simulink model "STEP3"  (R2020b)
settings: Solver=FixedStepDiscrete  StartTime=0.0  StopTime=inf  FixedStep=1  RelTol=1e-3  EnableMultiTasking=on
PreLoadFcn:
  | defaultRadioRequestMode = RadioRequestMode.OFF;
  | defaultCdRequestMode = CdRequestMode.EMPTY;
StartFcn:
  | clear sfcdplayerhelper;
  | sfcdplayergui;
StopFcn:
  | delete(sfcdplayergui);
model workspace (MATLAB code in the model file):
  | Ts = 0.01;  % setup system sample rate
settings Model: Creator=The MathWorks, Inc.  LastModifiedBy=Fong
settings DataIOCC: LimitDataPoints=on  SaveFormat=Array  SaveOutput=off  SaveTime=off  ReturnWorkspaceOutputs=off
settings OptimizationCC: DefaultParameterBehavior=Inlined  ExpressionDepthLimit=2147483647  StateBitsets=on  DataBitsets=on  ZeroExternalMemoryAtStartup=off  ZeroInternalMemoryAtStartup=off  InitFltsAndDblsToZero=on  EfficientFloat2IntCast=on  EfficientMapNaN2IntZero=off  LifeSpan=1  EfficientTunableParamExpr=on
settings DebuggingCC: UnderspecifiedInitializationDetection=Classic  MergeDetectMultiDrivingBlocksExec=none  FcnCallInpInsideContextMsg=warning  AllowSymbolicDim=off  StateNameClashWarn=warning  SFUnexpectedBacktrackingDiag=warning  SFNoUnconditionalDefaultTransitionDiag=warning  SFExecutionAtInitializationDiag=none  ArithmeticOperatorsInVariantConditions=warning
settings HardwareCC: ProdBitPerPointer=32  ProdBitPerSizeT=32  ProdBitPerPtrDiffT=32  ProdLargestAtomicFloat=None  ProdWordSize=32  ProdHWDeviceType=NEC->V850
settings ModelReferenceCC: ModelReferenceNumInstancesAllowed=Single  PropagateSignalLabelsOutOfModel=off
settings SFSimCC: SimUseLocalCustomCode=off  SimParseCustomCode=off  CustomCodeUndefinedFunction=UseInterfaceOnly
settings RTWCC: Description=Real-Time Workshop Embedded Coder (no auto configuration)  SystemTargetFile=ert.tlc  GenCodeOnly=on  TemplateMakefile=ert_default_tmf  GenerateReport=on  RTWUseLocalCustomCode=off  IncludeHyperlinkInReport=on  LaunchReport=on  GenerateTraceInfo=on  GenerateTraceReport=on  GenerateTraceReportSl=on  GenerateTraceReportSf=on  GenerateTraceReportEml=on
settings CodeAppCC: IgnoreCustomStorageClasses=off  CustomSymbolStrType=$N$R$M  CustomSymbolStrModelFcn=$N  StateflowObjectComments=on  InternalIdentifier=Classic
settings ERTTargetCC: MultiwordLength=2048  GenerateSampleERTMain=on  IncludeMdlTerminateFcn=off  SupportAbsoluteTime=off  PurelyIntegerCode=on  SupportNonFinite=off  SupportComplex=off  ERTCustomFileTemplate=example_file_process.tlc  ConvertIfToSwitch=off  SuppressUnreachableDefaultCases=off  EnableUserReplacementTypes=on
settings ConfigComp: CovMetricSettings=dw  CovSaveCumulativeToWorkspaceVar=on  CovSaveSingleToWorkspaceVar=on  CovExternalEMLEnable=off  CovSFcnEnable=off  DVMaxProcessTime=600  DVParameters=on  DVModelCoverageObjectives=MCDC  DVMaxTestCaseSteps=500  DVTestSuiteOptimization=CombinedObjectives  DVDetectActiveLogic=on  DVSaveHarnessModel=on  DVModelReferenceHarness=on  DVSaveReport=on  DVRebuildModelRepresentation=Always

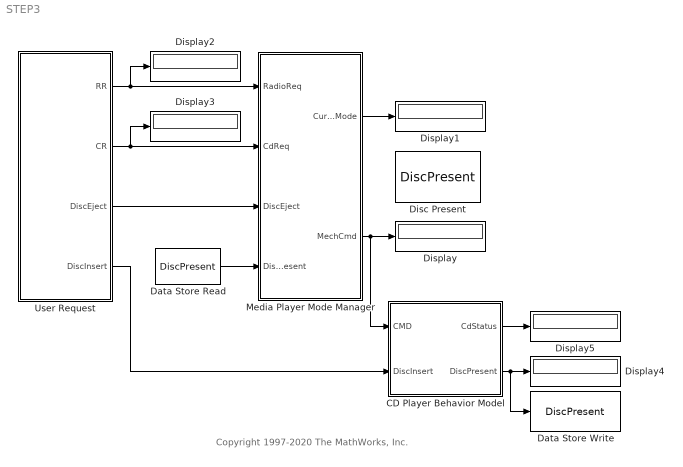
== system STEP3 ==
  note: Copyright 1997-2020 The MathWorks, Inc.
  CD Player Behavior Model : Stateflow chart  TreatAsAtomicUnit=on
  Data Store Read : DataStoreRead  DataStoreName=DiscPresent  SampleTime=0
  Data Store Write : DataStoreWrite  DataStoreName=DiscPresent
  Disc Present : DataStoreMemory  DataStoreName=DiscPresent  ShowAdditionalParam=off
  Display{,1..5} (6 alike) : Display
  Media Player Mode Manager : Stateflow chart  TreatAsAtomicUnit=on
  User Request : Stateflow chart  TreatAsAtomicUnit=on
  wires:
  User Request/2(CR) -> Media Player Mode Manager/2(CdReq), Display3/1
  Data Store Read/1 -> Media Player Mode Manager/4(DiscPresent)
  Media Player Mode Manager/2(MechCmd) -> Display/1, CD Player Behavior Model/1(CMD)
  Media Player Mode Manager/1(CurrentRadioMode) -> Display1/1
  User Request/1(RR) -> Media Player Mode Manager/1(RadioReq), Display2/1
  CD Player Behavior Model/1(CdStatus) -> Display5/1
  CD Player Behavior Model/2(" DiscPresent") -> Data Store Write/1, Display4/1
  User Request/4(DiscInsert) -> CD Player Behavior Model/2(DiscInsert)
  User Request/3(DiscEject) -> Media Player Mode Manager/3(DiscEject)

== stateflow chart STEP3/Media Player Mode Manager ==
  state ModeManager
    (history)
    state Standby
      entry: CurrentRadioMode = OFF;
      MechCmd = STOP;
    state ON
      (history)
      state CDMode
        en:
        CurrentRadioMode = CD;
        MechCmd = STOP;
        ex: MechCmd = STOP;
        state Play
          state Normal
            entry: MechCmd = PLAY;
          state Rew
            entry: MechCmd = REW;
          state FastForward
            entry: MechCmd = FF;
          (default) -> Normal
          Play -> Normal [order 3] : [CdReq == PLAY && !in(Normal)]
          Play -> Rew [order 2] : [CdReq == REW && !in(Rew)]
          Play -> FastForward [order 1] : [CdReq == FF && !in(FastForward)]
        state Stop
          entry: MechCmd = STOP;
        (default) -> Play [order 1] : [DiscPresent]
        (default) -> Stop [order 2]
        Play -> Stop [order 1] : [CdReq==STOP]
        Stop -> Play : [DiscPresent && CdReq==PLAY]
      state AMMode
        entry:
        CurrentRadioMode = AM;
        MechCmd = STOP;
      state FMMode
        entry:
        CurrentRadioMode = FM;
        MechCmd = STOP;
      (default) -> (junction 152)
      (junction 152) -> (junction 125)
      ON -> (junction 125) [order 1] : [hasChanged(RadioReq)]
      (junction 125) -> CDMode [order 1] : [RadioReq==CD]
      (junction 125) -> (junction 127) [order 2]
      (junction 127) -> AMMode [order 1] : [RadioReq==AM]
      (junction 127) -> (junction 128) [order 2]
      (junction 128) -> FMMode : /*RadioReq==FM*/
    (default) -> Standby
    Standby -> (junction 152) : [RadioReq != OFF]
    ON -> Standby [order 1] : [RadioReq == OFF]
  state Eject
    entry:
    MechCmd = EJECT;
  (default) -> ModeManager
  ModeManager -> Eject : [DiscEject]
  Eject -> ModeManager
  data: RadioReq input Enum: RadioRequestMode =0xFF; CdReq input Enum: CdRequestMode; DiscEject input; CurrentRadioMode output Enum: RadioRequestMode; DiscPresent input boolean; MechCmd output Enum: CdRequestMode

== stateflow chart STEP3/User Request ==
  (default) -> (junction 13) : {
      | RR = RadioRequestMode(ml.sfcdplayerhelper('get_radio_request'));
      | CR = CdRequestMode(ml.sfcdplayerhelper('get_cd_request'));
      | DiscInsert = ml.sfcdplayerhelper('get_insert_disc');
      | DiscEject = ml.sfcdplayerhelper('get_eject_disc');
      | }
  data: RR output Enum: RadioRequestMode; CR output Enum: CdRequestMode; DiscEject output boolean; DiscInsert output boolean

== stateflow chart STEP3/CD Player Behavior Model ==
  state Empty
    entry: CdStatus = EMPTY;
  state Inserting
    entry: CdStatus = DISCINSERT;
  state Ejecting
    entry: CdStatus = EJECT;
  state DiscPresent
    state STOP
      entry: CdStatus = STOP;
    state PLAY
      entry: CdStatus = PLAY;
    state FF
      entry: CdStatus = FF;
    state REW
      entry: CdStatus = REW;
    (default) -> STOP
    DiscPresent -> STOP [order 1] : [CMD == STOP]
    DiscPresent -> PLAY [order 2] : [CMD == PLAY]
    DiscPresent -> FF [order 4] : [CMD == FF]
    DiscPresent -> REW [order 3] : [CMD == REW]
  (default) -> Empty
  Ejecting -> Empty : after(1,sec)
  Empty -> Inserting : [DiscInsert]
  Inserting -> DiscPresent : after(1,sec)
  DiscPresent -> Ejecting [order 1] : [CMD == EJECT]
  data: CMD input; CdStatus output Enum: CdRequestMode; DiscInsert input boolean; DiscPresent output boolean
